simulink model "Simulaciones"  (R2024b)
settings: Solver=VariableStepAuto  StartTime=0.0  StopTime=60  RelTol=1e-3
values from neighbouring files (symbols this model uses):
  A = [0 0 1 0 ... (first row only)    [Sistema.m]
  B = [0 0;0 0;1/m 0;0 1/m]    [Sistema.m]
  C = eye(4)    [Sistema.m]
  Klqr = lqr(A,B,Q,R,0)    [Sistema.m]
  klqr = lqr(A,B,Q,R)    [Sistema.m]
  m = 2e3    (= 2000)    [Sistema.m]
  nr = (8-6.3)*1e5^2*ruido_m    (= 17000000000)    [Sistema.m]
  nrp = 1e4^2*ruido_m    (= 100000000)    [Sistema.m]
  nte = 1e-5^2*ruido_m    (= 1e-10)    [Sistema.m]
  ntep = 0.727e-5^2*ruido_m    (= 5.28529e-11)    [Sistema.m]
  pr = (9.6e7*0.01)^2*pertu_a    (= 921600000000)    [Sistema.m]
  pte = (0.23*0.01)^2*pertu_a    (= 5.29e-06)    [Sistema.m]
  R_k = diag([nr;nte;nrp;ntep^(1/2)])    [Sistema.m]
undefined symbols (not defined in the file or in its folder): Continuous, eta, K, K1, K2, Time, x_eq
libraries: ctrlSharedLib x1
settings Model: Creator=ricar  LastModifiedBy=ricar
settings RTWCC: GPUComputeCapability=3.5

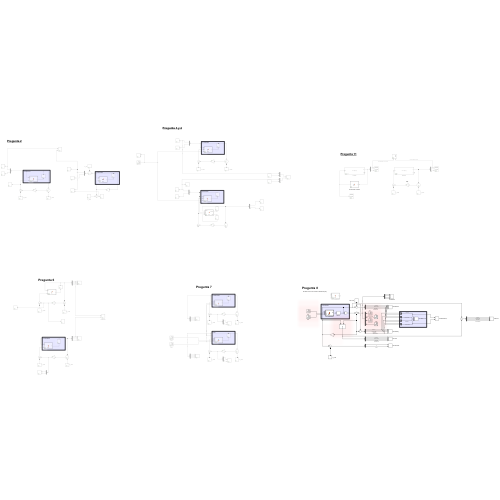
[thumbnail: Simulink's stored preview of the top-level diagram]
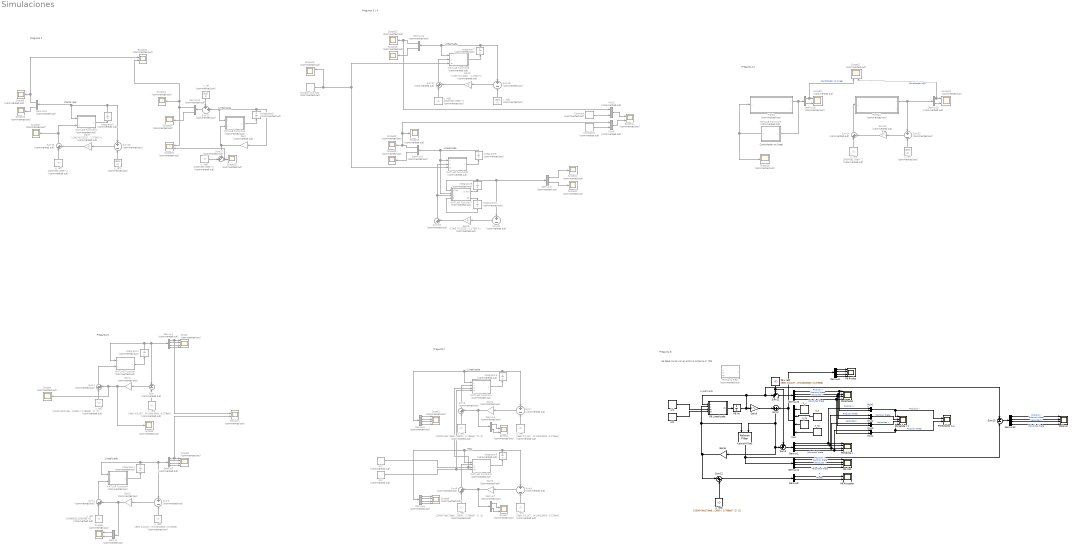
== system Simulaciones ==
  note: Se debe correr con el archivo sistema.m (P8)
  note: Pregunta 6
  note: Linealizada
  note: Linealizada
  note: Real
  note: Linealizada
  note: Pregunta 7
  note: Pregunta 8
  note: 8
  note: Controlador no lineal
  note: Pregunta 2
  note: Klqr
  note: Linealizada
  note: Linealizada
  note: Pregunta 3 y 4
  note: Linealizada
  note: Planta real
  note: Pregunta 11
  Ar1 : RandomNumber  Variance=pr  SampleTime=1e-4
  Ar2 : RandomNumber  Commented=on  Variance=(9.6e7*0.01)^2  SampleTime=1e-4
  At1 : RandomNumber  Variance=pte  SampleTime=1e-4
  At2 : RandomNumber  Commented=on  Variance=(0.24*0.01)^2  SampleTime=1e-4
  Constant : Constant  Commented=on  Value=6378e3
  Constant1 : Constant  Commented=on  Value=6378e3
  Demux{,4,7,13..19} (10 alike) : Demux  Commented=on  Outputs=2
  Demux{1,8,10..12} (5 alike) : Demux
  Demux{2..3,5..6} (4 alike) : Demux  Commented=on
  Demux9 : Demux  Outputs=2
  Gain : Gain  Commented=on  Gain=-Klqr  Multiplication=Matrix(K*u)
  Gain1 : Gain  Commented=on  Gain=-klqr  Multiplication=Matrix(K*u) (u vector)
  Gain10 : Gain  Commented=on  Gain=-K  Multiplication=Matrix(K*u)
  Gain2 : Gain  Commented=on  Gain=-klqr  Multiplication=Matrix(K*u)
  Gain3 : Gain  Gain=C  Multiplication=Matrix(K*u)
  Gain4 : Gain  Commented=on  Gain=-klqr  Multiplication=Matrix(K*u)
  Gain5 : Gain  Commented=on  Gain=-klqr  Multiplication=Matrix(K*u)
  Gain6 : Gain  Gain=-klqr  Multiplication=Matrix(K*u)
  Gain7 : Gain  Commented=on  Gain="-1.0e3 *[0.3225    1.1790]"  Multiplication=Matrix(K*u)
  Gain8 : Gain  Commented=on  Gain="-1.0e3 *[0.3225    1.1790]"  Multiplication=Matrix(K*u)
  Gain9 : Gain  Commented=on  Gain="-1.0e5 *[0.3225    1.1790]"  Multiplication=Matrix(K*u)
  Integrator1 : Integrator  Commented=on  InitialCondition=[8e6+2.0e6; 0;0;0]
  Integrator10 : Integrator  Commented=on  InitialCondition=eye(2)
  Integrator2 : Integrator  Commented=on  InitialCondition=[8e6+2.0e6; 0;0;0]
  Integrator3 : Integrator  Commented=on  InitialCondition=[8e6-1.5e6; -100]
  Integrator4 : Integrator  Commented=on  InitialCondition=[8e6; 0;0;1670*1000/3600 / 3.786e6]
  Integrator5 : Integrator  Commented=on  InitialCondition=[8e6; 0;0;1670*1000/3600 / 3.786e6]
  Integrator6 : Integrator  Commented=on  InitialCondition=[-1e6; 0]
  Integrator7 : Integrator  Commented=on  InitialCondition=[8e6; 0]
  Integrator8 : Integrator  Commented=on  InitialCondition=[8e6; 0]
  Integrator9 : Integrator  Commented=on  InitialCondition=[8e6; 0]
  Kalman Filter : ctrlSharedLib/Kalman Filter  TimeDomain=Continuous-Time  UseCurrentEstimator=on  ModelSource=Individual A, B, C, D matrices  ModelSourceVariable=ss(0.95,1,1,0,1)  A=A  B=B  C=C  D=0  NumberOfStates=1  NumberOfInputs=1  NumberOfOutputs=1  InitialEstimateSource=Dialog  X0=[0;0;0;0]  P0=10  UseK=off  UseGH=on  NumberOfProcessNoiseInputs=1  G=diag([1,1,1,1])  TimeInvariantG=on  H=eye(4)  TimeInvariantH=on  Q=Q_k  TimeInvariantQ=on  R=R_k  TimeInvariantR=on  N=0  TimeInvariantN=on  AddInputPort=on  AddEnablePort=off  OutputEstimatedY=off  OutputP=off  Ts=-1
  MATLAB Function : MATLAB Function  Commented=on  TreatAsAtomicUnit=on
  MATLAB Function1 : MATLAB Function  Commented=on  TreatAsAtomicUnit=on
  MATLAB Function2 : MATLAB Function  Commented=on  TreatAsAtomicUnit=on
  MATLAB Function3 : MATLAB Function  Commented=on  TreatAsAtomicUnit=on
  MATLAB Function4 : MATLAB Function  Commented=on  TreatAsAtomicUnit=on
  MATLAB Function5 : MATLAB Function  Commented=on  TreatAsAtomicUnit=on
  MATLAB Function6 : MATLAB Function  Commented=on  TreatAsAtomicUnit=on
  MATLAB Function7 : MATLAB Function  Commented=on  TreatAsAtomicUnit=on
  MATLAB Function8 : MATLAB Function  Commented=on  TreatAsAtomicUnit=on
  MATLAB Function9 : MATLAB Function  Commented=on  TreatAsAtomicUnit=on
  Mux : Mux
  Mux{1..4} (4 alike) : Mux  Inputs=2
  Mux5 : Mux  Commented=on  Inputs=2
  Mux6 : Mux  Commented=on  Inputs=2
  P8 Actuador : Scope  NumInputPorts=2
  P8 Error : Scope  NumInputPorts=4
  P8 Estados : Scope  NumInputPorts=4
  P8 Estados 1,4 : Scope  NumInputPorts=2
  P8 Int : Integrator  InitialCondition=[1.5e6; 0;1.5e6;6e-5]
  P8 Linealizada : MATLAB Function  TreatAsAtomicUnit=on
  P8 Salida Y X : Scope  NumInputPorts=4
  P8 Salida y : Scope  NumInputPorts=4
  P8 x ref1 : Constant  Value=[8e6; 0;0;1670*1000/3600 / 6.378e6]
  P8 xhat : Scope  NumInputPorts=4
  P9 Planta Real : MATLAB Function  Commented=on  TreatAsAtomicUnit=on
  P9 Ruidos : Scope  NumInputPorts=4
  Planta : Subsystem  Commented=on
      mask Display:
      | disp('\n\n\nẋ = f(x,u)\n\n\n')
      | port_label('input', 1, 'u');
      | port_label('output', 1, 'x');
      | port_label('output', 2, 'y');
  Planta1 : Subsystem  Commented=on
      mask Display:
      | disp('\n\n\nẋ = f(x,u)\n\n\n')
      | port_label('input', 1, 'u');
      | port_label('output', 1, 'x');
      | port_label('output', 2, 'y');
  Posicion : Scope  Commented=on  NumInputPorts=2
  Random Number : RandomNumber  Commented=on  Variance=(9.6e7)^2  SampleTime=1e-4
  Scope{,1,6,8} (4 alike) : Scope  Commented=on  NumInputPorts=4
  Scope{3..5,10..13,15,18,23..29} (16 alike) : Scope  Commented=on
  Scope{2,7,9,14,16..17,19..22} (10 alike) : Scope  Commented=on  NumInputPorts=2
  Sum{,5,7,9,16,18,20,22} (8 alike) : Sum  Commented=on  Inputs=+|-
  Sum{1,4,6,8,14..15,17,19} (8 alike) : Sum  Commented=on  Inputs=|++
  Sum10 : Sum  Inputs=+|-
  Sum11 : Sum  Inputs=++|
  Sum12 : Sum  Inputs=|++
  Sum13 : Sum  Commented=on  Inputs=++|
  Sum2 : Sum  Inputs=+|+
  Sum21 : Sum  Commented=on  Inputs=++|
  Sum3 : Sum  Inputs=++|
  n_r : RandomNumber  Variance=nr  SampleTime=1e-4
  n_rp : RandomNumber  Variance=nrp  SampleTime=1e-4
  n_t : RandomNumber  Variance=nte  SampleTime=1e-4
  n_tp : RandomNumber  Variance=ntep  SampleTime=1e-4
  u_ref1 : Constant  Commented=on  Value=[24999915.3593688 ;0]
  u_ref2 : Constant  Commented=on  Value=[2000*(8e17/8e6^2-8e6*(1670*1000/3600 / 3.786e6)^2) ;0]
  u_ref{3,7..9} (4 alike) : Constant  Commented=on  Value=2000*8e17/8e6^2
  u_ref4 : Constant  Commented=on  Value="[2000*(8e17/8e6^2-8e6*(1670*1000/3600 /  3.786e6)^2) ;0]"
  u_ref5 : Constant  Commented=on  Value="[2000*(8e17/8e6^2-8e6*(1670*1000/3600 /  3.786e6)^2) ;0]"
  u_ref6 : Constant  Value="[2000*(8e17/8e6^2-8e6*(1670*1000/3600 /  3.786e6)^2) ;0]"
  x_ref{,1,6..7} (4 alike) : Constant  Commented=on  Value=[8e6; 0]
  x_ref{2..5} (4 alike) : Constant  Commented=on  Value=[8e6; 0;0;1670*1000/3600 / 6.378e6]
  wires:
  Sum4/1 -> MATLAB Function4/2(u)
  u_ref1/1 -> Sum4/1
  Sum5/1 -> Gain2/1
  Gain2/1 -> Demux/1, Sum4/2
  x_ref2/1 -> Sum5/2
  MATLAB Function4/1(y) -> Integrator2/1
  u_ref2/1 -> Sum1/1
  Sum1/1 -> MATLAB Function/2(u)
  Integrator1/1 -> MATLAB Function/1(x), Demux2/1, Sum/1
  Demux2/2 -> Scope/2
  Demux2/3 -> Scope/3
  Demux2/4 -> Scope/4
  Gain1/1 -> Scope5/1, Scope4/1, Sum1/2
  MATLAB Function/1(y) -> Integrator1/1
  x_ref3/1 -> Sum/2
  Sum/1 -> Gain1/1
  Demux5/3 -> Scope8/3
  Demux5/4 -> Scope8/4
  Demux5/2 -> Scope8/2
  Demux5/1 -> Posicion/2, Scope8/1
  Integrator2/1 -> Sum5/1, Demux5/1, MATLAB Function4/1(x)
  Demux/1 -> Scope9/1
  Demux/2 -> Scope9/2
  Demux2/1 -> Posicion/1, Scope/1
  u_ref5/1 -> Sum6/1
  x_ref5/1 -> Sum7/2
  Gain4/1 -> Demux4/1, Sum6/2
  Demux3/4 -> Scope1/4
  Demux3/2 -> Scope1/2
  Sum7/1 -> Gain4/1
  Demux3/1 -> Scope1/1
  MATLAB Function1/1(y) -> Integrator4/1
  Integrator4/1 -> Sum7/1, MATLAB Function1/1(x), Demux3/1
  Demux3/3 -> Scope1/3
  Sum6/1 -> MATLAB Function1/2(u)
  Demux4/1 -> Scope2/1
  Demux4/2 -> Scope2/2
  Demux7/1 -> Scope7/1
  Demux7/2 -> Scope7/2
  u_ref4/1 -> Sum8/1
  Ar2/1 -> MATLAB Function1/3(ar), MATLAB Function2/3(ar)
  Sum8/1 -> MATLAB Function2/2(u)
  Demux6/3 -> Scope6/3
  Integrator5/1 -> Sum9/1, MATLAB Function2/1(x), Demux6/1
  Demux6/2 -> Scope6/2
  At2/1 -> MATLAB Function2/4(at), MATLAB Function1/4(at)
  Gain5/1 -> Demux7/1, Sum8/2
  x_ref4/1 -> Sum9/2
  Demux6/4 -> Scope6/4
  Sum9/1 -> Gain5/1
  Demux6/1 -> Scope6/1
  MATLAB Function2/1(y) -> Integrator5/1
  Gain3/1 -> Sum2/1
  Demux10/1 -> P8 Estados/1, Mux1/2  "Posicion r"
  Demux10/4 -> P8 Estados/4, Mux4/2  "Velocidad theta"
  Demux10/2 -> P8 Estados/2, Mux2/2  "Posicion theta"
  Demux10/3 -> P8 Estados/3, Mux3/2  "Velocidad r"
  P8 Linealizada/1(dx) -> P8 Int/1
  Mux/1 -> Demux8/1, Sum2/2
  n_r/1 -> Mux/1
  n_t/1 -> Mux/2
  n_rp/1 -> Mux/3
  n_tp/1 -> Mux/4
  Sum11/1 -> Demux10/1
  Gain6/1 -> Sum12/1, Kalman Filter/1, P8 Linealizada/2(u)
  Ar1/1 -> P8 Linealizada/3(ar)
  At1/1 -> P8 Linealizada/4(at)
  Demux1/1 -> P8 Salida y/1, Mux1/1  "Posicion r"
  Demux1/3 -> P8 Salida y/3, Mux3/1  "Velocidad r"
  Demux1/2 -> P8 Salida y/2, Mux2/1  "Posicion theta"
  Demux1/4 -> P8 Salida y/4, Mux4/1  "Velocidad theta"
  Demux9/2 -> P8 Actuador/2  "Ftheta"
  Demux9/1 -> P8 Actuador/1  "Fr"
  Sum2/1 -> Sum3/2, Gain6/1, Kalman Filter/2
  Sum3/1 -> Demux1/1
  P8 x ref1/1 -> Sum3/1, Sum11/1
  Mux1/1 -> P8 Salida Y X/1, P8 Estados 1,4/1  "Posicion r"
  Mux2/1 -> P8 Salida Y X/2  "Posicion theta"
  Mux3/1 -> P8 Salida Y X/3  "Velocidad r"
  Mux4/1 -> P8 Estados 1,4/2, P8 Salida Y X/4  "Posicion theta"
  Demux8/1 -> P9 Ruidos/1
  Demux8/2 -> P9 Ruidos/2
  Demux8/3 -> P9 Ruidos/3
  Demux8/4 -> P9 Ruidos/4
  Kalman Filter/1 -> Demux11/1, Sum10/2
  Demux11/1 -> P8 xhat/1  "Posicion r"
  Demux11/3 -> P8 xhat/3  "Velocidad r"
  Demux11/4 -> P8 xhat/4  "Velocidad theta"
  Demux11/2 -> P8 xhat/2  "Posicion theta"
  Demux12/3 -> P8 Error/3  "Velocidad r"
  Demux12/4 -> P8 Error/4  "Velocidad theta"
  Demux12/1 -> P8 Error/1  "Posicion r"
  Demux12/2 -> P8 Error/2  "Posicion theta"
  Sum10/1 -> Demux12/1
  P8 Int/1 -> P8 Linealizada/1(x), Sum10/1, Sum11/2, Gain3/1
  Sum12/1 -> Demux9/1
  u_ref6/1 -> Sum12/2
  Demux19/2 -> Scope22/2
  Gain8/1 -> Sum17/2
  MATLAB Function8/1(y) -> Integrator8/1
  Sum19/1 -> MATLAB Function8/2(u), MATLAB Function7/3(u)
  u_ref9/1 -> Sum14/1
  Integrator7/1 -> Sum18/1, MATLAB Function6/1(x), Demux14/1
  Constant/1 -> Mux5/2
  Demux17/2 -> Scope11/1
  Integrator6/1 -> Gain/1, Sum13/2, MATLAB Function5/1(x)
  MATLAB Function6/1(y) -> Integrator7/1
  Planta/1(x) -> Demux18/1, MATLAB Function9/1(x)
  Sum13/1 -> Demux15/1
  MATLAB Function7/1(dxhat) -> Integrator9/1
  Mux6/1 -> Scope14/2
  Sum17/1 -> MATLAB Function6/2(u)
  Sum21/1 -> Scope16/2, Scope15/1
  MATLAB Function3/1(y) -> Integrator3/1
  Constant1/1 -> Mux6/2
  Gain10/1 -> Sum14/2
  Demux15/1 -> Scope24/1, Scope20/2, Scope16/1
  Integrator3/1 -> Sum16/1, MATLAB Function3/1(x), Demux13/1
  u_ref3/1 -> Sum17/1
  Sum18/1 -> Gain8/1
  MATLAB Function7/2(dP) -> Integrator10/1
  Gain7/1 -> Sum15/2
  u_ref8/1 -> Sum21/2
  Integrator8/1 -> MATLAB Function7/2(x), MATLAB Function8/1(x), Demux16/1
  Demux13/2 -> Scope10/1
  Sum22/1 -> Gain10/1
  x_ref6/1 -> Sum18/2
  u_ref7/1 -> Sum15/1
  Integrator10/1 -> MATLAB Function7/4(P)
  Mux5/1 -> Scope14/1
  Demux17/1 -> Scope12/1
  Demux14/1 -> Scope23/1, Mux5/1
  Gain9/1 -> Sum19/2
  Demux18/1 -> Scope21/1, Scope17/1  "Controlador no lineal"
  Demux16/2 -> Scope29/1
  x_ref/1 -> Sum13/1
  Planta1/1(x) -> Sum22/1, Demux19/1
  Sum15/1 -> Scope27/1, MATLAB Function3/2(u)
  Gain/1 -> MATLAB Function5/2(u), Sum21/1
  Integrator9/1 -> Sum20/1, Demux17/1, MATLAB Function7/1(xhat)
  MATLAB Function5/1(y) -> Integrator6/1
  x_ref7/1 -> Sum22/2
  Sum16/1 -> Gain7/1
  Demux16/1 -> Scope13/1, Mux6/1, Scope28/1
  MATLAB Function9/1(u) -> Planta/1(u), Scope18/1
  Demux13/1 -> Scope20/1, Scope3/1
  Demux15/2 -> Scope25/1
  x_ref1/1 -> Sum16/2
  Demux19/1 -> Scope21/2, Scope22/1  "Controlador LQR"
  Sum14/1 -> Planta1/1(u)
  Random Number/1 -> Scope19/1, MATLAB Function6/3(ar), MATLAB Function8/3(ar)
  Demux18/2 -> Scope17/2
  Sum20/1 -> Gain9/1
  Demux14/2 -> Scope26/1

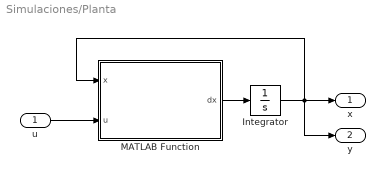
== system Simulaciones/Planta ==
  u : Inport
  Integrator : Integrator  InitialCondition=[8.3e6; -2e4]
  MATLAB Function : MATLAB Function  TreatAsAtomicUnit=on
  x : Outport
  y : Outport  Port=2
  wires:
  MATLAB Function/1(dx) -> Integrator/1
  Integrator/1 -> y/1, x/1, MATLAB Function/1(x)
  u/1 -> MATLAB Function/2(u)

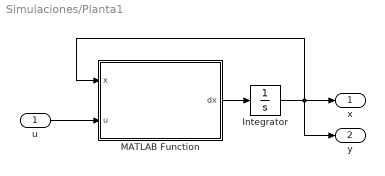
== system Simulaciones/Planta1 ==
  u : Inport
  Integrator : Integrator  InitialCondition=[8.3e6; -2e4]
  MATLAB Function : MATLAB Function  TreatAsAtomicUnit=on
  x : Outport
  y : Outport  Port=2
  wires:
  MATLAB Function/1(dx) -> Integrator/1
  Integrator/1 -> y/1, x/1, MATLAB Function/1(x)
  u/1 -> MATLAB Function/2(u)

== matlab function Simulaciones/MATLAB Function7 ==
  data: xhat input; x input; u input; dxhat output; P input; dP output
function [dxhat,dP] = fcn(xhat,x,u,P)

A = [0 1; 2*8e17/8e6^3 0];
B = [0;1/2000];
C = eye(2);

L = [0    0
    0    316230];

x_ref = [8e6; 0];
u_ref = 2000*8e17/8e6^2;

Q_k = 1*[0, 9.6e7];                  % Ruido de proceso
R_k = 1e-6*[1 1];                  % Ruido de medicion

%Filtro de Kalman
dxhat_t = A*(xhat-x_ref) + B*(u-u_ref) + L*(C*x - C*xhat);
P = A*P*A'+Q_k;
e = xhat - x;
K = P*C'*inv(C*P*C'+R_k);
dxhat = dxhat_t - K*e;
dP = K*C*P;

== matlab function Simulaciones/MATLAB Function8 ==
  data: x input; u input; y output; ar input
function y = fcn(x,u,ar)
A = [0 1; 2*8e17/8e6^3 0];
B = [0;1/2000];
%C = eye(2);

x_ref = [8e6; 0];
u_ref = 2000*8e17/8e6^2;

if x(1) <= 6378e3
    dx = [0;0];
else
dx = A*(x-x_ref) + B*(u-u_ref)+[0;1]*ar;
end


y = dx;

== matlab function Simulaciones/MATLAB Function9 ==
  data: x input; u output; m parameter; eta parameter; x_eq parameter; K1 parameter; K2 parameter
function u = fcn(x, m, eta, x_eq, K1, K2)
    
    u = m * ((-K1 * x(2)) - (x(1) - x_eq(1)) + (eta/x(1)^2) -K2 * (x(2) + K1 * (x(1) - x_eq(1))));

== matlab function Simulaciones/Planta/MATLAB Function ==
  data: x input; u input; dx output; eta parameter; m parameter
function dx = fcn(x, u, eta, m)

    dx = zeros(2,1);
    dx(1) = x(2);
    dx(2) = -(eta/x(1)^2) + (u/m);

end

== matlab function Simulaciones/Planta1/MATLAB Function ==
  data: x input; u input; dx output; eta parameter; m parameter
function dx = fcn(x, u, eta, m)

    dx = zeros(2,1);
    dx(1) = x(2);
    dx(2) = -(eta/x(1)^2) + (u/m);

end

== matlab function Simulaciones/MATLAB Function1 ==
  data: x input; u input; y output; ar input; at input
function y = fcn(x,u,ar,at)
m = 2e3; %m
mu = 8e17; %m3/s2
r_ref = 8e6; %m
theta_tierra = 1670*1000/3600 / 6.378e6; %m/s
%Para la trayectoria definida:

fr = m*(mu/r_ref^2-r_ref*theta_tierra^2);
ftheta = 0;

A = [0 0 1 0;
     0 0 0 1;
     2*mu/r_ref^3+theta_tierra^2, 2*r_ref*theta_tierra 0 0
     0 0 -2*theta_tierra/r_ref 0];

B = [0 0;0 0;1/m 0;0 1/m];
%C = eye(2);

x_ref = [8e6; 0; 0 ; theta_tierra];
u_ref = [fr;ftheta];

if x(1) <= 6.378e6
    y = zeros(size(A,1),1);
else
    y = A*(x-x_ref) + B*(u-u_ref) +[0;0;ar;at];
end

== matlab function Simulaciones/MATLAB Function ==
  data: x input; u input; y output
function y = fcn(x,u)

m = 2e3; %m
mu = 8e17; %m3/s2
%Para la trayectoria definida:
xz = x;
uz = u;

if xz(1) <= 6.378e6
    dx = zeros(4,1);
else
    dx = [xz(3);
          xz(4);
          -mu/(xz(1))^2+xz(1)*xz(4)^2+1/m*uz(1);
          -2*xz(3)*xz(4)/(xz(1)) + 1/m*uz(2)];
end


y = dx;

== matlab function Simulaciones/MATLAB Function2 ==
  data: x input; u input; y output; ar input; at input
function y = fcn(x,u,ar,at)

m = 2e3; %m
mu = 8e17; %m3/s2
%Para la trayectoria definida:
xz = x;
uz = u;

if xz(1) <= 6.378e6
    dx = zeros(4,1);
else
    dx = [xz(3);
          xz(4);
          -mu/(xz(1))^2+xz(1)*xz(4)^2+1/m*uz(1)+ar;
          -2*xz(3)*xz(4)/(xz(1)) + 1/m*uz(2)+at];
end


y = dx;

== matlab function Simulaciones/P9 Planta Real ==
  data: x input; u input; y output; ar input; at input
function y = fcn(x,u,ar,at)

m = 2e3; %m
mu = 8e17; %m3/s2
%Para la trayectoria definida:
xz = x;
uz = u;

if xz(1) <= 6.378e6
    dx = zeros(4,1);
else
    dx = [xz(3);
          xz(4);
          -mu/(xz(1))^2+xz(1)*xz(4)^2+1/m*uz(1)+ar;
          -2*xz(3)*xz(4)/(xz(1)) + 1/m*uz(2)+at];
end


y = dx;

== matlab function Simulaciones/MATLAB Function4 ==
  data: x input; u input; y output
function y = fcn(x,u)
m = 2e3; %m
mu = 8e17; %m3/s2
r_ref = 8e6; %m
theta_tierra = 1670*1000/3600 / 6.378e6; %m/s
%Para la trayectoria definida:

fr = m*(mu/r_ref^2-r_ref*theta_tierra^2);
ftheta = 0;

A = [0 0 1 0;
     0 0 0 1;
     2*mu/r_ref^3+theta_tierra^2, 2*r_ref*theta_tierra 0 0
     0 0 -2*theta_tierra/r_ref 0];

B = [0 0;0 0;1/m 0;0 1/m];
%C = eye(2);

x_ref = [8e6; 0; 0 ; theta_tierra];
u_ref = [fr;ftheta];

if x(1) <= 6.378e6
    y = zeros(size(A,1),1);
else
    y = A*(x-x_ref) + B*(u-u_ref);
end

== matlab function Simulaciones/P8 Linealizada ==
  data: x input; u input; ar input; at input; dx output
function dx = fcn(x,u,ar,at)
m = 2e3; %m
mu = 8e17; %m3/s2
r_ref = 8e6; %m
theta_tierra = 1670*1000/3600 / 6.378e6; %m/s
%Para la trayectoria definida:

A = [0 0 1 0;
     0 0 0 1;
     2*mu/r_ref^3+theta_tierra^2, 2*r_ref*theta_tierra 0 0
     0 0 -2*theta_tierra/r_ref 0];

B = [0 0;0 0;1/m 0;0 1/m];

if x(1) <= 6.378e6-8e6
    dx = zeros(size(A,1),1);
else
    dx = A*x + B*u +[0;0;ar;at];
end

== matlab function Simulaciones/MATLAB Function3 ==
  data: x input; u input; y output
function y = fcn(x,u)

if x(1) <= 6378e3
    dx = [0;0];
else
dx = [x(2);-8e17/(x(1))^2+u/2000];
end


y = dx;

== matlab function Simulaciones/MATLAB Function5 ==
  data: x input; u input; y output
function y = fcn(x,u)
A = [0 1; 2*8e17/8e6^3 0];
B = [0;1/2000];
%C = eye(2);

x_ref = [8e6; 0];
u_ref = 2000*8e17/8e6^2;

if x(1) <= 6378e3 -8e6
    dx = [0;0];
else
dx = A*x + B*u;
end


y = dx;

== matlab function Simulaciones/MATLAB Function6 ==
  data: x input; u input; y output; ar input
function y = fcn(x,u,ar)
A = [0 1; 2*8e17/8e6^3 0];
B = [0;1/2000];
%C = eye(2);

x_ref = [8e6; 0];
u_ref = 2000*8e17/8e6^2;

if x(1) <= 6378e3
    dx = [0;0];
else
dx = A*(x-x_ref) + B*(u-u_ref)+[0;1]*ar;
end


y = dx;
